simulink library "wind3D_cl"  (R2020a)
settings: Solver=VariableStepAuto  StartTime=0.0  StopTime=10.0  RelTol=1e-3
undefined symbols (not defined in the file): Env, PLANT
libraries: AirDensity_ul x1, LinWindVel3D_ul x1, stopSim_ul x1
settings Model: Creator=jbore  LastModifiedBy=John Jr
settings SFSimCC: CustomCodeUndefinedFunction=UseInterfaceOnly

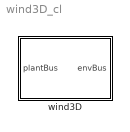
== system wind3D_cl ==
  wind3D : Subsystem  VariantControl=strcmpi(PLANT,'wind3D')

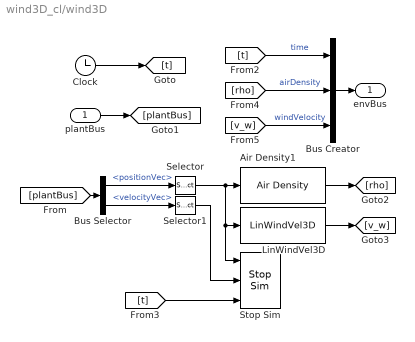
== system wind3D_cl/wind3D ==
  plantBus : Inport
  Air Density1 : AirDensity_ul/Air Density  rho=Env.density.Value  g=Env.grav.Value  M=Env.M.Value  R=Env.R.Value  T_0=Env.temp.Value
  Bus Creator : BusCreator  Inputs=3
  Bus Selector : BusSelector  OutputSignals=positionVec,velocityVec
  Clock : Clock
  LinWindVel3D : LinWindVel3D_ul/LinWindVel3D
  Selector : Selector  InputPortWidth=3  IndexOptions=Index vector (dialog)  Indices=3  OutputSizes=1
  Selector1 : Selector  InputPortWidth=3  IndexOptions=Index vector (dialog)  Indices=3  OutputSizes=1
  Stop Sim : stopSim_ul/Stop Sim  z_0=0  t_b=Veh.motor.burnTime.Value
  envBus : Outport  VectorParamsAs1DForOutWhenUnconnected=off
  wires:
  [t] -> Stop Sim/3
  Selector1/1 -> Stop Sim/2
  Bus Selector/2 -> Selector1/1  "<velocityVec>"
  Selector/1 -> Air Density1/1, LinWindVel3D/1, Stop Sim/1
  Bus Selector/1 -> Selector/1  "<positionVec>"
  Bus Creator/1 -> envBus/1
  Clock/1 -> [t]
  [t] -> Bus Creator/1  "time"
  plantBus/1 -> [plantBus]
  [plantBus] -> Bus Selector/1
  Air Density1/1 -> [rho]
  [rho] -> Bus Creator/2  "airDensity"
  LinWindVel3D/1 -> [v_w]
  [v_w] -> Bus Creator/3  "windVelocity"
